simulink model "player_ball_7_8players3_2_withoutlidar"  (R2021b)
settings: Solver=VariableStepAuto  StartTime=0.0  StopTime=300  RelTol=1e-3
model workspace (MAT data in the model file):
  trailfuzzy = 'trailfuzzy.fis'
values from neighbouring files (symbols this model uses):
  initBallPos = fieldCenter    [robotSoccerParams.m]
  robotDetectorMaxHits = 5    [robotSoccerParams.m]
  sampleTime = 0.05    [robotSoccerParams.m]
undefined symbols (not defined in the file or in its folder): DiscIntNeverNeededParam
libraries: mobileRoboticsLib x45, dspindex x15, fuzblock x9
(part 1 of 2)
settings Model: NumberOfSteps=10  Creator=kstkr  LastModifiedBy=kstkr
settings DebuggingCC: AlgebraicLoopMsg=none

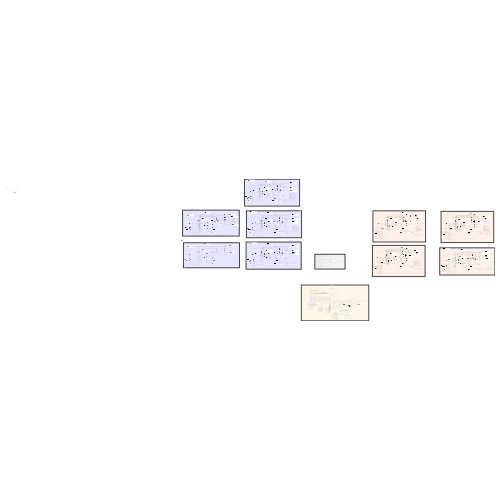
[thumbnail: Simulink's stored preview of the top-level diagram]
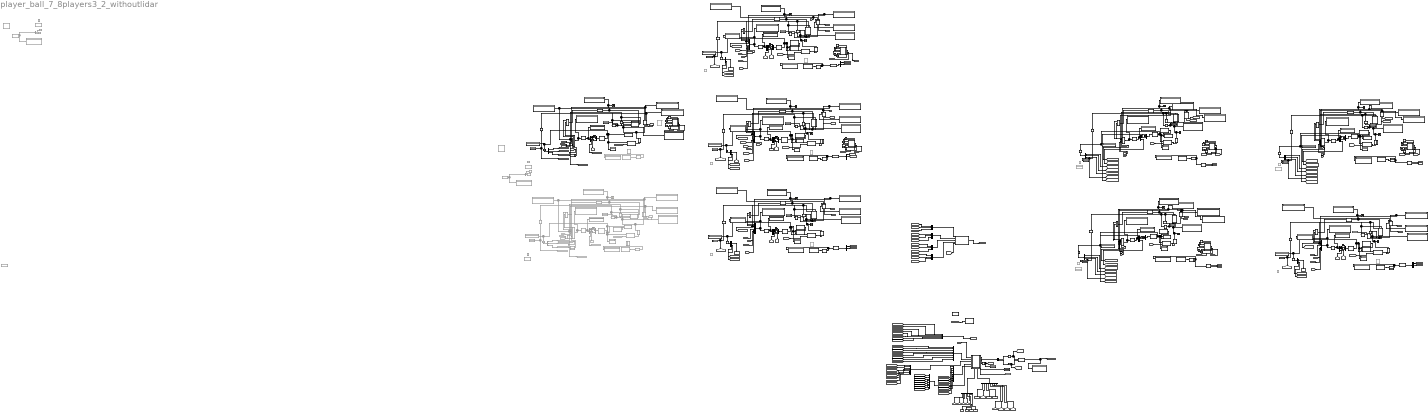
== system player_ball_7_8players3_2_withoutlidar ==
  note: EMOTIONS
  note: Subsystem1
  note: Subsystem1
  note: Ensure the sensor parameters point to the same variables.
  note: Checks team possession and ball held
  note: change mf to sinesoidal
  note: check for postition 80,10
  note: Subsystem1
  note: change mf to sinesoidal
  note: check for postition 80,10
  note: Subsystem1
  note: Ensure the sensor parameters point to the same variables.
  note: Attackert2_1
  note: Ensure the sensor parameters point to the same variables.
  note: Attackert2_2
  note: Ensure the sensor parameters point to the same variables.
  note: defendert2
  note: Ensure the sensor parameters point to the same variables.
  note: Subsystem1
  note: Ensure the sensor parameters point to the same variables.
  note: defentert2_1
  note: Ensure the sensor parameters point to the same variables.
  Add Constant{,1..3} (4 alike) : Bias  Commented=on  Bias=0.3
  Ball Dynamics : MATLAB Function  Commented=on  TreatAsAtomicUnit=on
  Ball Dynamics1 : MATLAB Function  Commented=on  TreatAsAtomicUnit=on
  Ball Dynamics2 : MATLAB Function  Commented=on  TreatAsAtomicUnit=on
  Ball Dynamics3 : MATLAB Function  Commented=on  TreatAsAtomicUnit=on
  Ball Dynamics4 : MATLAB Function  Commented=on  TreatAsAtomicUnit=on
  Ball Dynamics5 : MATLAB Function  Commented=on  TreatAsAtomicUnit=on
  Ball Dynamics6 : MATLAB Function  Commented=on  TreatAsAtomicUnit=on
  Bus Creator{,1..6} (7 alike) : BusCreator  Inputs=8
  Chart3 : Stateflow chart  TreatAsAtomicUnit=on
      settings: PortSchema="{\"entries\":[{\"content\":{\"sides\":[{\"content\":{\"connectorIds\":[\"In1\",\"In2\",\"In3\",\"In4\",\"In6\"]},\"type\":\"ConnectorPlacement.EquallySpacedRectSide\",\"uuid\":\"100227f9-96df-4219-ace2-0d84d12d506e\"},{\"content\":{\"connectorIds\":[\"Out1\",\"Out2\",\"Out3\",\"Out4\"],\"side\":\"RIGHT\"},\"type\":\"ConnectorPlacement.EquallySpacedRectSide\",\"uuid\":\"5179a9f1-5caf-4bf7-8381-53191773d399\"},{\"content\":{\"connectorIds\":[],\"side\":\"TOP\"},\"type\":\"ConnectorPlacement.EquallySpacedRectSide\",\"uuid\":\"b02881a3-df96-4ac6-93d3-ffe2a0056366\"},{\"content\":{\"connectorIds\":[\"In7\",\"In5\"],\"side\":\"BOTTOM\"},\"type\":\"ConnectorPlacement.EquallySpacedRectSide\",\"uuid\":\"6df5f698-3dd3-4c11-801f-bca33302808b\"}]},\"type\":\"ConnectorPlacement.EquallySpacedConnector\",\"uuid\":\"a5fc3484-c51e-4d4d-931a-fb20b747c02a\"}],\"packageUris\":[\"http://schema.mathworks.com/mf0/Connector/R2020b\"],\"version\":\"1.0\"}"
  Constant{,1..9} (10 alike) : Constant  Commented=on  Value=0.5
  Demux{,2,6..10,12..24,26..33} (28 alike) : Demux  Outputs=3
  Demux1 : Demux  Commented=on  Outputs=3
  Demux11 : Demux  Outputs=2
  Demux25 : Demux  Commented=on  Outputs=2
  Demux3 : Demux  Commented=on  Outputs=3
  Demux4 : Demux  Commented=on  Outputs=2
  Demux5 : Demux  Commented=on  Outputs=3
  Display{,1,3,6..9,11,13..24,31..41,43..96} (85 alike) : Display
  Display{2,4..5,10,12,25..30,42} (12 alike) : Display  Commented=on
  From29 : From  Commented=on  GotoTag=objPoses
  From30 : From  Commented=on  GotoTag=rPose_y3
  From31 : From  Commented=on  GotoTag=rPose_theta3
  From32 : From  Commented=on  GotoTag=rPose_y3
  From33 : From  Commented=on  GotoTag=teamHeld
  From34 : From  Commented=on  GotoTag=rPose_x3
  From35 : From  Commented=on  GotoTag=rPose_x3
  Generic Vehicle Simulation : mobileRoboticsLib/Utilities/Generic Vehicle Simulation  initX=25  initY=28  initAngle=0  Ts=sampleTime
      settings: SourceProductName=Mobile Robotics Simulation Toolbox
  Generic Vehicle Simulation1 : mobileRoboticsLib/Utilities/Generic Vehicle Simulation  Commented=on  initX=30  initY=50  initAngle=0  Ts=sampleTime
      settings: SourceProductName=Mobile Robotics Simulation Toolbox
  Generic Vehicle Simulation2 : mobileRoboticsLib/Utilities/Generic Vehicle Simulation  initX=25  initY=15  initAngle=0  Ts=sampleTime
      settings: SourceProductName=Mobile Robotics Simulation Toolbox
  Generic Vehicle Simulation3 : mobileRoboticsLib/Utilities/Generic Vehicle Simulation  initX=2  initY=30  initAngle=0  Ts=sampleTime
      settings: SourceProductName=Mobile Robotics Simulation Toolbox
  Generic Vehicle Simulation4 : mobileRoboticsLib/Utilities/Generic Vehicle Simulation  initX=60  initY=40  initAngle=pi  Ts=sampleTime
      settings: SourceProductName=Mobile Robotics Simulation Library
  Generic Vehicle Simulation5 : mobileRoboticsLib/Utilities/Generic Vehicle Simulation  initX=60  initY=20  initAngle=pi  Ts=sampleTime
      settings: SourceProductName=Mobile Robotics Simulation Library
  Generic Vehicle Simulation6 : mobileRoboticsLib/Utilities/Generic Vehicle Simulation  initX=75  initY=30  initAngle=pi  Ts=sampleTime
      settings: SourceProductName=Mobile Robotics Simulation Library
  Generic Vehicle Simulation7 : mobileRoboticsLib/Utilities/Generic Vehicle Simulation  initX=88  initY=30  initAngle=pi  Ts=sampleTime
      settings: SourceProductName=Mobile Robotics Simulation Toolbox
  Generic Vehicle Simulation8 : mobileRoboticsLib/Utilities/Generic Vehicle Simulation  initX=15  initY=45  initAngle=0  Ts=sampleTime
      settings: SourceProductName=Mobile Robotics Simulation Toolbox
  Goal Range{,1,3..5} (5 alike) : Display
  Goal Range2 : Display  Commented=on
  GoalLeftAngle{,1,3..5} (5 alike) : Display
  GoalLeftAngle2 : Display  Commented=on
  Goto19 : Goto  Commented=on  GotoTag=ballHeld3
  Goto20 : Goto  Commented=on  GotoTag=KickPower3
  Goto21 : Goto  Commented=on  GotoTag=rPose_x3
  Goto22 : Goto  Commented=on  GotoTag=rPose_y3
  Goto23 : Goto  Commented=on  GotoTag=rPose_theta3
  Goto24 : Goto  Commented=on  GotoTag=robotIdx3
  Goto25 : Goto  Commented=on  GotoTag=ballVel3
  Ground{,2..8} (8 alike) : Ground
  Ground1 : Ground  Commented=on
  IC{1,4,10,13,16,19,22,25} (8 alike) : InitialCondition
  IC{2..3,5..6,11..12,14..15,17..18,20..21,23..24,26..27} (16 alike) : InitialCondition  Value=0
  IC7 : InitialCondition  Commented=on
  IC8 : InitialCondition  Commented=on  Value=0
  IC9 : InitialCondition  Commented=on  Value=0
  MATLAB Function : MATLAB Function  TreatAsAtomicUnit=on
  MATLAB Function1 : MATLAB Function  Commented=on  TreatAsAtomicUnit=on
  MATLAB Function10 : MATLAB Function  TreatAsAtomicUnit=on
  MATLAB Function11 : MATLAB Function  TreatAsAtomicUnit=on
  MATLAB Function12 : MATLAB Function  TreatAsAtomicUnit=on
  MATLAB Function2 : MATLAB Function  TreatAsAtomicUnit=on
  MATLAB Function3 : MATLAB Function  Commented=on  TreatAsAtomicUnit=on
  MATLAB Function4 : MATLAB Function  TreatAsAtomicUnit=on
  MATLAB Function5 : MATLAB Function  TreatAsAtomicUnit=on
  MATLAB Function6 : MATLAB Function  TreatAsAtomicUnit=on
  MATLAB Function7 : MATLAB Function  TreatAsAtomicUnit=on
  MATLAB Function8 : MATLAB Function  TreatAsAtomicUnit=on
  MATLAB Function9 : MATLAB Function  TreatAsAtomicUnit=on
  Memory{,3..4,7..11} (8 alike) : Memory  InitialCondition=[15 2 0]  InheritSampleTime=on
  Memory1 : Memory  InheritSampleTime=on
  Memory{12,16,20,24,28,32} (6 alike) : Memory  InitialCondition=5  InheritSampleTime=on
  Memory{13,15,17,19,21,23,25,27,29,31,33,35} (12 alike) : Memory  InitialCondition=2  InheritSampleTime=on
  Memory{14,18,22,26,30,34} (6 alike) : Memory  InitialCondition=8  InheritSampleTime=on
  Memory2 : Memory  Commented=on  InitialCondition=[15 2 0]  InheritSampleTime=on
  Memory5 : Memory  InheritSampleTime=on  LinearizeAsDelay=on
  Memory6 : Memory  InheritSampleTime=on  LinearizeAsDelay=on
  Multi-Robot Environment : mobileRoboticsLib/Environments/Multi-Robot Environment  numRobots=8  mapName=map  showWaypoints=off  showObjects=on  objectColors=objColors  objectMarkers=objMarkers  showRobotIds=on  plotSensorLines=on
      settings: SourceProductName=Mobile Robotics Simulation Toolbox
  Multi-Robot Lidar Sensor2 : mobileRoboticsLib/Environments/Multi-Robot Lidar Sensor  robotIdx=2  mapName=map  sensorOffset=[0,0]  scanAngles=[-pi/4 0 pi/4]  maxRange=5
      settings: SourceProductName=Mobile Robotics Simulation Toolbox
  Multi-Robot Lidar Sensor3 : mobileRoboticsLib/Environments/Multi-Robot Lidar Sensor  Commented=on  robotIdx=3  mapName=map  sensorOffset=[0,0]  scanAngles=[-pi/4 0 pi/4]  maxRange=5
      settings: SourceProductName=Mobile Robotics Simulation Toolbox
  Multi-Robot Lidar Sensor4 : mobileRoboticsLib/Environments/Multi-Robot Lidar Sensor  robotIdx=4  mapName=map  sensorOffset=[0,0]  scanAngles=[-pi/4 0 pi/4]  maxRange=5
      settings: SourceProductName=Mobile Robotics Simulation Toolbox
  Multi-Robot Lidar Sensor5 : mobileRoboticsLib/Environments/Multi-Robot Lidar Sensor  robotIdx=5  mapName=map  sensorOffset=[0,0]  scanAngles=[-pi/4 0 pi/4]  maxRange=5
      settings: SourceProductName=Mobile Robotics Simulation Toolbox
  Multi-Robot Lidar Sensor6 : mobileRoboticsLib/Environments/Multi-Robot Lidar Sensor  robotIdx=6  mapName=map  sensorOffset=[0,0]  scanAngles=[-pi/4 0 pi/4]  maxRange=5
      settings: SourceProductName=Mobile Robotics Simulation Toolbox
  Multi-Robot Lidar Sensor7 : mobileRoboticsLib/Environments/Multi-Robot Lidar Sensor  robotIdx=7  mapName=map  sensorOffset=[0,0]  scanAngles=[-pi/4 0 pi/4]  maxRange=5
      settings: SourceProductName=Mobile Robotics Simulation Toolbox
  Multi-Robot Lidar Sensor8 : mobileRoboticsLib/Environments/Multi-Robot Lidar Sensor  robotIdx=8  mapName=map  sensorOffset=[0,0]  scanAngles=[-pi/4 0 pi/4]  maxRange=5
      settings: SourceProductName=Mobile Robotics Simulation Toolbox
  Multi-Robot Lidar Sensor9 : mobileRoboticsLib/Environments/Multi-Robot Lidar Sensor  robotIdx=3  mapName=map  sensorOffset=[0,0]  scanAngles=[-pi/4 0 pi/4]  maxRange=5
      settings: SourceProductName=Mobile Robotics Simulation Toolbox
  Multi-Robot Visualizer : mobileRoboticsLib/Environments/Multi-Robot Visualizer  idx=1  radius=1  robotColor=[0 0 1]  showTraj=on  hasLidar=off  sensorOffset=[0,0]  scanAngles=[-pi/4 0 pi/4]  maxNumScans=0  hasObjDetector=off  objDetectorOffset=[0,0]  objDetectorAngle=0  objDetectorFOV=pi/3  objDetectorMaxRange=5  hasRobotDetector=off  robotDetectorOffset=[0,0]  robotDetectorAngle=0  robotDetectorFOV=pi/3  robotDetectorMaxRange=5  robotDetectorNumDetections=0
      settings: SourceProductName=Mobile Robotics Simulation Toolbox
  Multi-Robot Visualizer1 : mobileRoboticsLib/Environments/Multi-Robot Visualizer  Commented=on  idx=3  radius=1  robotColor=[0 0 1]  showTraj=on  hasLidar=on  sensorOffset=[0,0]  scanAngles=[-pi/4 0 pi/4]  maxNumScans=0  hasObjDetector=off  objDetectorOffset=[0,0]  objDetectorAngle=0  objDetectorFOV=pi/3  objDetectorMaxRange=5  hasRobotDetector=off  robotDetectorOffset=[0,0]  robotDetectorAngle=0  robotDetectorFOV=pi/3  robotDetectorMaxRange=5  robotDetectorNumDetections=0
      settings: SourceProductName=Mobile Robotics Simulation Toolbox
  Multi-Robot Visualizer2 : mobileRoboticsLib/Environments/Multi-Robot Visualizer  idx=2  radius=1  robotColor=[0 0 1]  showTraj=on  hasLidar=on  sensorOffset=[0,0]  scanAngles=[-pi/4 0 pi/4]  maxNumScans=0  hasObjDetector=off  objDetectorOffset=[0,0]  objDetectorAngle=0  objDetectorFOV=pi/3  objDetectorMaxRange=5  hasRobotDetector=off  robotDetectorOffset=[0,0]  robotDetectorAngle=0  robotDetectorFOV=pi/3  robotDetectorMaxRange=5  robotDetectorNumDetections=0
      settings: SourceProductName=Mobile Robotics Simulation Toolbox
  Multi-Robot Visualizer3 : mobileRoboticsLib/Environments/Multi-Robot Visualizer  idx=4  radius=1  robotColor=[0 0 1]  showTraj=on  hasLidar=on  sensorOffset=[0,0]  scanAngles=[-pi/4 0 pi/4]  maxNumScans=0  hasObjDetector=off  objDetectorOffset=[0,0]  objDetectorAngle=0  objDetectorFOV=pi/3  objDetectorMaxRange=5  hasRobotDetector=off  robotDetectorOffset=[0,0]  robotDetectorAngle=0  robotDetectorFOV=pi/3  robotDetectorMaxRange=5  robotDetectorNumDetections=0
      settings: SourceProductName=Mobile Robotics Simulation Toolbox
  Multi-Robot Visualizer4 : mobileRoboticsLib/Environments/Multi-Robot Visualizer  idx=5  radius=1  robotColor=[1 0 0]  showTraj=on  hasLidar=on  sensorOffset=[0,0]  scanAngles=[-pi/4 0 pi/4]  maxNumScans=0  hasObjDetector=off  objDetectorOffset=[0,0]  objDetectorAngle=0  objDetectorFOV=pi/3  objDetectorMaxRange=5  hasRobotDetector=off  robotDetectorOffset=[0,0]  robotDetectorAngle=0  robotDetectorFOV=pi/3  robotDetectorMaxRange=5  robotDetectorNumDetections=0
      settings: SourceProductName=Mobile Robotics Simulation Toolbox
  Multi-Robot Visualizer5 : mobileRoboticsLib/Environments/Multi-Robot Visualizer  idx=6  radius=1  robotColor=[1 0 0]  showTraj=on  hasLidar=on  sensorOffset=[0,0]  scanAngles=[-pi/4 0 pi/4]  maxNumScans=0  hasObjDetector=off  objDetectorOffset=[0,0]  objDetectorAngle=0  objDetectorFOV=pi/3  objDetectorMaxRange=5  hasRobotDetector=off  robotDetectorOffset=[0,0]  robotDetectorAngle=0  robotDetectorFOV=pi/3  robotDetectorMaxRange=5  robotDetectorNumDetections=0
      settings: SourceProductName=Mobile Robotics Simulation Toolbox
  Multi-Robot Visualizer6 : mobileRoboticsLib/Environments/Multi-Robot Visualizer  idx=7  radius=1  robotColor=[1 0 0]  showTraj=on  hasLidar=on  sensorOffset=[0,0]  scanAngles=[-pi/4 0 pi/4]  maxNumScans=0  hasObjDetector=off  objDetectorOffset=[0,0]  objDetectorAngle=0  objDetectorFOV=pi/3  objDetectorMaxRange=5  hasRobotDetector=off  robotDetectorOffset=[0,0]  robotDetectorAngle=0  robotDetectorFOV=pi/3  robotDetectorMaxRange=5  robotDetectorNumDetections=0
      settings: SourceProductName=Mobile Robotics Simulation Toolbox
  Multi-Robot Visualizer7 : mobileRoboticsLib/Environments/Multi-Robot Visualizer  idx=8  radius=1  robotColor=[1 0 0]  showTraj=on  hasLidar=on  sensorOffset=[0,0]  scanAngles=[-pi/4 0 pi/4]  maxNumScans=0  hasObjDetector=off  objDetectorOffset=[0,0]  objDetectorAngle=0  objDetectorFOV=pi/3  objDetectorMaxRange=5  hasRobotDetector=off  robotDetectorOffset=[0,0]  robotDetectorAngle=0  robotDetectorFOV=pi/3  robotDetectorMaxRange=5  robotDetectorNumDetections=0
      settings: SourceProductName=Mobile Robotics Simulation Toolbox
  Multi-Robot Visualizer8 : mobileRoboticsLib/Environments/Multi-Robot Visualizer  idx=3  radius=1  robotColor=[0 0 1]  showTraj=on  hasLidar=on  sensorOffset=[0,0]  scanAngles=[-pi/4 0 pi/4]  maxNumScans=0  hasObjDetector=off  objDetectorOffset=[0,0]  objDetectorAngle=0  objDetectorFOV=pi/3  objDetectorMaxRange=5  hasRobotDetector=off  robotDetectorOffset=[0,0]  robotDetectorAngle=0  robotDetectorFOV=pi/3  robotDetectorMaxRange=5  robotDetectorNumDetections=0
      settings: SourceProductName=Mobile Robotics Simulation Toolbox
  Mux{,4,6,8,10,12,14,16,18..21} (12 alike) : Mux  Inputs=3
  Mux1 : Mux  Commented=on  Inputs=3
  Mux11 : Mux  Inputs=9
  Mux13 : Mux  Inputs=9
  Mux15 : Mux  Inputs=8
  Mux17 : Mux  Inputs=10
  Mux2 : Mux  Inputs=10
  Mux3 : Mux  Commented=on  Inputs=10
  Mux5 : Mux  Inputs=10
  Mux7 : Mux  Inputs=8
  Mux9 : Mux  Inputs=9
  Object Detections [range, angle, label]{,2..8} (8 alike) : Display
  "Object Detections [range, angle, label]1" : Display  Commented=on
  Object Detector{,2..8} (8 alike) : mobileRoboticsLib/Environments/Object Detector  mapName=map  sensorOffset=objDetectorOffset  sensorAngle=objDetectorAngle  fieldOfView=objDetectorFOV  maxRange=objDetectorRange  maxDetections=objDetectorMaxHits  sampleTime=-1
      Object Detector settings: SourceProductName=Mobile Robotics Simulation Toolbox
      Object Detector2 settings: SourceProductName=Mobile Robotics Simulation Toolbox
      Object Detector3 settings: SourceProductName=Mobile Robotics Simulation Toolbox
      Object Detector4 settings: SourceProductName=Ground Vehicles Library
      Object Detector5 settings: SourceProductName=Ground Vehicles Library
      Object Detector6 settings: SourceProductName=Ground Vehicles Library
      Object Detector7 settings: SourceProductName=Mobile Robotics Simulation Toolbox
      Object Detector8 settings: SourceProductName=Mobile Robotics Simulation Toolbox
  Object Detector1 : mobileRoboticsLib/Environments/Object Detector  Commented=on  mapName=map  sensorOffset=objDetectorOffset  sensorAngle=objDetectorAngle  fieldOfView=objDetectorFOV  maxRange=objDetectorRange  maxDetections=objDetectorMaxHits  sampleTime=-1
      settings: SourceProductName=Mobile Robotics Simulation Toolbox
  "Objects [x, y, label]1" : Constant  Commented=on  Value=[45, 30, 1; 0,15,2; 0, 45, 2; 90, 15, 3; 90, 45, 3]
  "Objects [x, y, label]2" : Constant  Commented=on  Value=[45, 30, 1; 0,15,2; 0, 45, 2; 90, 15, 3; 90, 45, 3]
  Package Objects Array1 : Subsystem
  Plot Soccer Field : MATLAB Function  TreatAsAtomicUnit=on
  Robot Detector1 : mobileRoboticsLib/Environments/Robot Detector  Commented=on  mapName=map  robotIdx=1  sensorOffset=robotDetectorOffset  sensorAngle=robotDetectorAngle  sensorFOV=2*pi  maxRange=100  maxDetections=robotDetectorMaxHits  sampleTime=sampleTime
      link override Robot Detector: mapName=map  maxDetections=5
      settings: SourceProductName=Mobile Robotics Simulation Toolbox
  Robot Detector2 : mobileRoboticsLib/Environments/Robot Detector  mapName=map  robotIdx=2  sensorOffset=robotDetectorOffset  sensorAngle=robotDetectorAngle  sensorFOV=2*pi  maxRange=100  maxDetections=robotDetectorMaxHits  sampleTime=sampleTime
      link override Robot Detector: mapName=map  maxDetections=5
      settings: SourceProductName=Mobile Robotics Simulation Toolbox
  Robot Detector3 : mobileRoboticsLib/Environments/Robot Detector  Commented=on  mapName=map  robotIdx=3  sensorOffset=robotDetectorOffset  sensorAngle=robotDetectorAngle  sensorFOV=2*pi  maxRange=100  maxDetections=robotDetectorMaxHits  sampleTime=sampleTime
      link override Robot Detector: mapName=map  maxDetections=5
      settings: SourceProductName=Mobile Robotics Simulation Toolbox
  Robot Detector4 : mobileRoboticsLib/Environments/Robot Detector  mapName=map  robotIdx=4  sensorOffset=robotDetectorOffset  sensorAngle=robotDetectorAngle  sensorFOV=2*pi  maxRange=100  maxDetections=robotDetectorMaxHits  sampleTime=sampleTime
      link override Robot Detector: mapName=map  maxDetections=5
      settings: SourceProductName=Mobile Robotics Simulation Toolbox
  Robot Detector5 : mobileRoboticsLib/Environments/Robot Detector  mapName=map  robotIdx=5  sensorOffset=robotDetectorOffset  sensorAngle=robotDetectorAngle  sensorFOV=pi/3  maxRange=100  maxDetections=robotDetectorMaxHits  sampleTime=sampleTime
      link override Robot Detector: mapName=map  maxDetections=5
      settings: SourceProductName=Mobile Robotics Simulation Toolbox
  Robot Detector6 : mobileRoboticsLib/Environments/Robot Detector  mapName=map  robotIdx=6  sensorOffset=robotDetectorOffset  sensorAngle=robotDetectorAngle  sensorFOV=pi/3  maxRange=100  maxDetections=robotDetectorMaxHits  sampleTime=sampleTime
      link override Robot Detector: mapName=map  maxDetections=5
      settings: SourceProductName=Mobile Robotics Simulation Toolbox
  Robot Detector7 : mobileRoboticsLib/Environments/Robot Detector  mapName=map  robotIdx=7  sensorOffset=robotDetectorOffset  sensorAngle=robotDetectorAngle  sensorFOV=pi/3  maxRange=100  maxDetections=robotDetectorMaxHits  sampleTime=sampleTime
      link override Robot Detector: mapName=map  maxDetections=5
      settings: SourceProductName=Mobile Robotics Simulation Toolbox
  Robot Detector8 : mobileRoboticsLib/Environments/Robot Detector  mapName=map  robotIdx=8  sensorOffset=robotDetectorOffset  sensorAngle=robotDetectorAngle  sensorFOV=2*pi  maxRange=100  maxDetections=robotDetectorMaxHits  sampleTime=sampleTime
      link override Robot Detector: mapName=map  maxDetections=5
      settings: SourceProductName=Mobile Robotics Simulation Toolbox
  Robot Detector9 : mobileRoboticsLib/Environments/Robot Detector  mapName=map  robotIdx=3  sensorOffset=robotDetectorOffset  sensorAngle=robotDetectorAngle  sensorFOV=2*pi  maxRange=100  maxDetections=robotDetectorMaxHits  sampleTime=sampleTime
      link override Robot Detector: mapName=map  maxDetections=5
      settings: SourceProductName=Mobile Robotics Simulation Toolbox
  Scope{,1,4,6,8,10,12,14} (8 alike) : Scope
  Scope{3,5,7,9,11,13,15} (7 alike) : Scope  NumInputPorts=2
  Scope2 : Scope  Commented=on
  Variable Selector{,3..8,10..14} (12 alike) : dspindex/Variable Selector  NumInputs=1  rowsOrCols=Rows  IdxMode=Fixed  Elements="[1  ]"  ZerOneIdxMode=One-based  errmode=Clip Index  FillMode=off  FillValues=0
  Variable Selector1 : dspindex/Variable Selector  Commented=on  NumInputs=1  rowsOrCols=Rows  IdxMode=Fixed  Elements="[1  ]"  ZerOneIdxMode=One-based  errmode=Clip Index  FillMode=off  FillValues=0
  Variable Selector2 : dspindex/Variable Selector  Commented=on  NumInputs=1  rowsOrCols=Columns  IdxMode=Fixed  Elements=[1 2]  ZerOneIdxMode=One-based  errmode=Clip Index  FillMode=on  FillValues=0
  Variable Selector9 : dspindex/Variable Selector  Commented=on  NumInputs=1  rowsOrCols=Columns  IdxMode=Fixed  Elements=[1 2]  ZerOneIdxMode=One-based  errmode=Clip Index  FillMode=on  FillValues=0
  Zero Pad Detections1 : MATLAB Function  Commented=on  TreatAsAtomicUnit=on  mask(Zero Pad Detections){maxHits=robotDetectorMaxHits}
      mask prompts: maxHits "Maximum Sensor Hits"
      mask help: Zero pads detections matrix so it is fixed-size and works with arrays of buses.
  Zero Pad Detections10 : MATLAB Function  TreatAsAtomicUnit=on  mask(Zero Pad Detections){maxHits=robotDetectorMaxHits}
      mask prompts: maxHits "Maximum Sensor Hits"
      mask help: Zero pads detections matrix so it is fixed-size and works with arrays of buses.
  Zero Pad Detections11 : MATLAB Function  Commented=on  TreatAsAtomicUnit=on  mask(Zero Pad Detections){maxHits=robotDetectorMaxHits}
      mask prompts: maxHits "Maximum Sensor Hits"
      mask help: Zero pads detections matrix so it is fixed-size and works with arrays of buses.
  Zero Pad Detections12 : MATLAB Function  TreatAsAtomicUnit=on  mask(Zero Pad Detections){maxHits=robotDetectorMaxHits}
      mask prompts: maxHits "Maximum Sensor Hits"
      mask help: Zero pads detections matrix so it is fixed-size and works with arrays of buses.
  Zero Pad Detections13 : MATLAB Function  TreatAsAtomicUnit=on  mask(Zero Pad Detections){maxHits=robotDetectorMaxHits}
      mask prompts: maxHits "Maximum Sensor Hits"
      mask help: Zero pads detections matrix so it is fixed-size and works with arrays of buses.
  Zero Pad Detections14 : MATLAB Function  TreatAsAtomicUnit=on  mask(Zero Pad Detections){maxHits=robotDetectorMaxHits}
      mask prompts: maxHits "Maximum Sensor Hits"
      mask help: Zero pads detections matrix so it is fixed-size and works with arrays of buses.
  Zero Pad Detections15 : MATLAB Function  TreatAsAtomicUnit=on  mask(Zero Pad Detections){maxHits=robotDetectorMaxHits}
      mask prompts: maxHits "Maximum Sensor Hits"
      mask help: Zero pads detections matrix so it is fixed-size and works with arrays of buses.
  Zero Pad Detections16 : MATLAB Function  TreatAsAtomicUnit=on  mask(Zero Pad Detections){maxHits=robotDetectorMaxHits}
      mask prompts: maxHits "Maximum Sensor Hits"
      mask help: Zero pads detections matrix so it is fixed-size and works with arrays of buses.
  Zero Pad Detections17 : MATLAB Function  TreatAsAtomicUnit=on  mask(Zero Pad Detections){maxHits=robotDetectorMaxHits}
      mask prompts: maxHits "Maximum Sensor Hits"
      mask help: Zero pads detections matrix so it is fixed-size and works with arrays of buses.
  Zero Pad Detections18 : MATLAB Function  TreatAsAtomicUnit=on  mask(Zero Pad Detections){maxHits=robotDetectorMaxHits}
      mask prompts: maxHits "Maximum Sensor Hits"
      mask help: Zero pads detections matrix so it is fixed-size and works with arrays of buses.
  Zero Pad Detections19 : MATLAB Function  TreatAsAtomicUnit=on  mask(Zero Pad Detections){maxHits=robotDetectorMaxHits}
      mask prompts: maxHits "Maximum Sensor Hits"
      mask help: Zero pads detections matrix so it is fixed-size and works with arrays of buses.
  Zero Pad Detections2 : MATLAB Function  Commented=on  TreatAsAtomicUnit=on  mask(Zero Pad Detections){maxHits=robotDetectorMaxHits}
      mask prompts: maxHits "Maximum Sensor Hits"
      mask help: Zero pads detections matrix so it is fixed-size and works with arrays of buses.
  Zero Pad Detections20 : MATLAB Function  Commented=on  TreatAsAtomicUnit=on  mask(Zero Pad Detections){maxHits=robotDetectorMaxHits}
      mask prompts: maxHits "Maximum Sensor Hits"
      mask help: Zero pads detections matrix so it is fixed-size and works with arrays of buses.
  Zero Pad Detections21 : MATLAB Function  TreatAsAtomicUnit=on  mask(Zero Pad Detections){maxHits=robotDetectorMaxHits}
      mask prompts: maxHits "Maximum Sensor Hits"
      mask help: Zero pads detections matrix so it is fixed-size and works with arrays of buses.
  Zero Pad Detections22 : MATLAB Function  TreatAsAtomicUnit=on  mask(Zero Pad Detections){maxHits=robotDetectorMaxHits}
      mask prompts: maxHits "Maximum Sensor Hits"
      mask help: Zero pads detections matrix so it is fixed-size and works with arrays of buses.
  Zero Pad Detections23 : MATLAB Function  Commented=on  TreatAsAtomicUnit=on  mask(Zero Pad Detections){maxHits=robotDetectorMaxHits}
      mask prompts: maxHits "Maximum Sensor Hits"
      mask help: Zero pads detections matrix so it is fixed-size and works with arrays of buses.
  Zero Pad Detections24 : MATLAB Function  TreatAsAtomicUnit=on  mask(Zero Pad Detections){maxHits=robotDetectorMaxHits}
      mask prompts: maxHits "Maximum Sensor Hits"
      mask help: Zero pads detections matrix so it is fixed-size and works with arrays of buses.
  Zero Pad Detections3 : MATLAB Function  Commented=on  TreatAsAtomicUnit=on  mask(Zero Pad Detections){maxHits=robotDetectorMaxHits}
      mask prompts: maxHits "Maximum Sensor Hits"
      mask help: Zero pads detections matrix so it is fixed-size and works with arrays of buses.
  Zero Pad Detections4 : MATLAB Function  TreatAsAtomicUnit=on  mask(Zero Pad Detections){maxHits=robotDetectorMaxHits}
      mask prompts: maxHits "Maximum Sensor Hits"
      mask help: Zero pads detections matrix so it is fixed-size and works with arrays of buses.
  Zero Pad Detections5 : MATLAB Function  TreatAsAtomicUnit=on  mask(Zero Pad Detections){maxHits=robotDetectorMaxHits}
      mask prompts: maxHits "Maximum Sensor Hits"
      mask help: Zero pads detections matrix so it is fixed-size and works with arrays of buses.
  Zero Pad Detections6 : MATLAB Function  Commented=on  TreatAsAtomicUnit=on  mask(Zero Pad Detections){maxHits=robotDetectorMaxHits}
      mask prompts: maxHits "Maximum Sensor Hits"
      mask help: Zero pads detections matrix so it is fixed-size and works with arrays of buses.
  Zero Pad Detections7 : MATLAB Function  TreatAsAtomicUnit=on  mask(Zero Pad Detections){maxHits=robotDetectorMaxHits}
      mask prompts: maxHits "Maximum Sensor Hits"
      mask help: Zero pads detections matrix so it is fixed-size and works with arrays of buses.
  Zero Pad Detections8 : MATLAB Function  Commented=on  TreatAsAtomicUnit=on  mask(Zero Pad Detections){maxHits=robotDetectorMaxHits}
      mask prompts: maxHits "Maximum Sensor Hits"
      mask help: Zero pads detections matrix so it is fixed-size and works with arrays of buses.
  Zero Pad Detections9 : MATLAB Function  Commented=on  TreatAsAtomicUnit=on  mask(Zero Pad Detections){maxHits=robotDetectorMaxHits}
      mask prompts: maxHits "Maximum Sensor Hits"
      mask help: Zero pads detections matrix so it is fixed-size and works with arrays of buses.
  ball : MATLAB Function  TreatAsAtomicUnit=on
  ball1 : MATLAB Function  TreatAsAtomicUnit=on
  ball2 : MATLAB Function  TreatAsAtomicUnit=on
  ball3 : MATLAB Function  Commented=on  TreatAsAtomicUnit=on
  ball4 : MATLAB Function  TreatAsAtomicUnit=on
  ball5 : MATLAB Function  TreatAsAtomicUnit=on
  ball6 : MATLAB Function  TreatAsAtomicUnit=on
  ball7 : MATLAB Function  TreatAsAtomicUnit=on
  ball8 : MATLAB Function  TreatAsAtomicUnit=on
  idx3 goal_range_angles : MATLAB Function  TreatAsAtomicUnit=on
  idx3 goal_range_angles1 : MATLAB Function  TreatAsAtomicUnit=on
  idx3 goal_range_angles2 : MATLAB Function  TreatAsAtomicUnit=on
  idx3 goal_range_angles3 : MATLAB Function  Commented=on  TreatAsAtomicUnit=on
  idx3 goal_range_angles4 : MATLAB Function  TreatAsAtomicUnit=on
  idx3 goal_range_angles5 : MATLAB Function  TreatAsAtomicUnit=on
  idx3 goal_range_angles6 : MATLAB Function  TreatAsAtomicUnit=on
  idx3 goal_range_angles7 : MATLAB Function  TreatAsAtomicUnit=on
  idx3 goal_range_angles8 : MATLAB Function  TreatAsAtomicUnit=on
  robot_actions1 : fuzblock/Fuzzy Logic  Controller  FIS='A1trialfuzzyball6_2.fis'  OutputSampleNumber=101  DataType=double  FuzzifiedInputs=off  RuleFiringStrengths=off  RuleOutputs=off  AggregatedOutputs=off  SimulateUsing=Interpreted execution  OutOfRangeInputValueMessage=warning  NoRuleFiredMessage=warning  EmptyOutputFuzzySetMessage=warning
  robot_actions2 : fuzblock/Fuzzy Logic  Controller  Commented=on  FIS='A1trialfuzzyball6_2.fis'  OutputSampleNumber=101  DataType=double  FuzzifiedInputs=off  RuleFiringStrengths=off  RuleOutputs=off  AggregatedOutputs=off  SimulateUsing=Interpreted execution  OutOfRangeInputValueMessage=warning  NoRuleFiredMessage=warning  EmptyOutputFuzzySetMessage=warning
  robot_actions3 : fuzblock/Fuzzy Logic  Controller  FIS='D1trialfuzzyball6_1_1.fis'  OutputSampleNumber=101  DataType=double  FuzzifiedInputs=off  RuleFiringStrengths=off  RuleOutputs=off  AggregatedOutputs=off  SimulateUsing=Interpreted execution  OutOfRangeInputValueMessage=warning  NoRuleFiredMessage=warning  EmptyOutputFuzzySetMessage=warning
  robot_actions4 : fuzblock/Fuzzy Logic  Controller  FIS='G1trialfuzzyball4.fis'  OutputSampleNumber=101  DataType=double  FuzzifiedInputs=off  RuleFiringStrengths=off  RuleOutputs=off  AggregatedOutputs=off  SimulateUsing=Interpreted execution  OutOfRangeInputValueMessage=warning  NoRuleFiredMessage=warning  EmptyOutputFuzzySetMessage=warning
  robot_actions5 : fuzblock/Fuzzy Logic  Controller  FIS='A1trialfuzzyball3_1.fis'  OutputSampleNumber=101  DataType=double  FuzzifiedInputs=off  RuleFiringStrengths=off  RuleOutputs=off  AggregatedOutputs=off  SimulateUsing=Interpreted execution  OutOfRangeInputValueMessage=warning  NoRuleFiredMessage=warning  EmptyOutputFuzzySetMessage=warning
  robot_actions6 : fuzblock/Fuzzy Logic  Controller  FIS='A1trialfuzzyball3_1.fis'  OutputSampleNumber=101  DataType=double  FuzzifiedInputs=off  RuleFiringStrengths=off  RuleOutputs=off  AggregatedOutputs=off  SimulateUsing=Interpreted execution  OutOfRangeInputValueMessage=warning  NoRuleFiredMessage=warning  EmptyOutputFuzzySetMessage=warning
  robot_actions7 : fuzblock/Fuzzy Logic  Controller  FIS='A1trialfuzzyball3_1.fis'  OutputSampleNumber=101  DataType=double  FuzzifiedInputs=off  RuleFiringStrengths=off  RuleOutputs=off  AggregatedOutputs=off  SimulateUsing=Interpreted execution  OutOfRangeInputValueMessage=warning  NoRuleFiredMessage=warning  EmptyOutputFuzzySetMessage=warning
  robot_actions8 : fuzblock/Fuzzy Logic  Controller  FIS='G2trialfuzzyball4.fis'  OutputSampleNumber=101  DataType=double  FuzzifiedInputs=off  RuleFiringStrengths=off  RuleOutputs=off  AggregatedOutputs=off  SimulateUsing=Interpreted execution  OutOfRangeInputValueMessage=warning  NoRuleFiredMessage=warning  EmptyOutputFuzzySetMessage=warning
  robot_actions9 : fuzblock/Fuzzy Logic  Controller  FIS='D1trialfuzzyball6_2_1.fis'  OutputSampleNumber=101  DataType=double  FuzzifiedInputs=off  RuleFiringStrengths=off  RuleOutputs=off  AggregatedOutputs=off  SimulateUsing=Interpreted execution  OutOfRangeInputValueMessage=warning  NoRuleFiredMessage=warning  EmptyOutputFuzzySetMessage=warning
  wires:
  Robot Detector1/1 -> Zero Pad Detections2/1(u)
  Zero Pad Detections2/1(y) -> Display5/1  "robotDetections"
  Mux/1 -> Generic Vehicle Simulation/1
  Ground/1 -> Mux/2
  robot_actions1/1 -> Display13/1, Demux/1  "v"
  Demux/1 -> [ballVel1], Mux/1
  Demux/2 -> Mux/3
  Generic Vehicle Simulation/1 -> Display11/1, Memory/1, Display/1, Object Detector/1, Multi-Robot Visualizer/1  "pose"
  Mux2/1 -> Display3/1, robot_actions1/1
  Object Detector/1 -> Zero Pad Detections4/1(u)  "detections"
  Variable Selector/1 -> Demux2/1
  Demux2/1 -> Mux2/2
  [objPoses] -> Multi-Robot Environment/1
  Demux2/2 -> Mux2/1
  Zero Pad Detections4/1(y) -> ball/1(u), "Object Detections [range, angle, label]"/1, idx3 goal_range_angles/1(u)  "robotDetections"
  ball/1(y) -> Scope/1, Display9/1, Variable Selector/1
  idx3 goal_range_angles/1(goalRight_angle) -> Mux2/4, Display6/1
  idx3 goal_range_angles/2(goalRange) -> Goal Range/1, Mux2/5
  idx3 goal_range_angles/3(goalLeft_angle) -> Mux2/6, GoalLeftAngle/1
  Variable Selector2/1 -> Demux4/1, Display10/1
  Demux4/1 -> Add Constant/1
  Demux4/2 -> Add Constant1/1
  Memory/1 -> Demux6/1
  Demux6/1 -> [rPose_x1]
  Demux6/2 -> [rPose_y1]
  Demux6/3 -> [rPose_theta1]
  Demux/3 -> [KickPower1]
  ball/3(robotIdx) -> IC1/1, IC2/1
  IC1/1 -> [robotIdx1], Display15/1
  ball/2(ballHeld) -> [ballHeld1], Mux2/3, IC3/1
  IC2/1 -> Display14/1, ball/3("robotIdx ")
  IC3/1 -> ball/2("ballHeld ")
  IC6/1 -> Display18/1, ball1/2("ballHeld ")
  IC5/1 -> ball1/3("robotIdx ")
  ball1/2(ballHeld) -> IC6/1, [ballHeld2], Mux5/3
  IC4/1 -> Display19/1, [robotIdx2]
  ball1/3(robotIdx) -> IC5/1, IC4/1
  Demux7/3 -> [KickPower2]
  Demux10/3 -> [rPose_theta2]
  Demux10/2 -> [rPose_y2]
  Demux10/1 -> [rPose_x2]
  Memory4/1 -> Demux10/1
  idx3 goal_range_angles1/3(goalLeft_angle) -> GoalLeftAngle1/1
  idx3 goal_range_angles1/2(goalRange) -> Mux5/4, Goal Range1/1
  idx3 goal_range_angles1/1(goalRight_angle) -> [leftpoleangle2], Display22/1
  ball1/1(y) -> Variable Selector3/1, Display23/1, Scope1/1
  Zero Pad Detections7/1(y) -> "Object Detections [range, angle, label]2"/1, ball1/1(u), idx3 goal_range_angles1/1(u), Scope3/1  "robotDetections"
  Demux8/2 -> Mux5/1
  Multi-Robot Lidar Sensor2/1 -> Multi-Robot Visualizer2/2
  Demux8/1 -> Mux5/2
  Variable Selector3/1 -> Demux8/1
  Object Detector2/1 -> Zero Pad Detections7/1(u)  "detections"
  Mux5/1 -> robot_actions3/1, Display16/1, Display20/1
  Generic Vehicle Simulation2/1 -> Multi-Robot Visualizer2/1, Display7/1, Object Detector2/1, Memory4/1, Display8/1  "pose"
  Demux7/2 -> Mux4/3
  Demux7/1 -> [ballVel2], Mux4/1
  robot_actions3/1 -> Demux7/1, Display17/1  "v"
  Ground2/1 -> Mux4/2
  Mux4/1 -> Generic Vehicle Simulation2/1
  Zero Pad Detections5/1(y) -> Variable Selector4/1, Display21/1  "robotDetections"
  Robot Detector2/1 -> Zero Pad Detections5/1(u)
  [objPoses] -> Object Detector/2
  [objPoses] -> Object Detector2/2
  Demux9/2 -> [rdet_angle]
  Demux9/1 -> [rdet_range]
  [rdet_range] -> Mux5/5
  [rdet_angle] -> Mux5/6
  Variable Selector4/1 -> Demux9/1
  Chart3/1(ballPose) -> Demux11/1
  [rPose_theta2] -> Bus Creator6/2
  [rPose_theta1] -> Bus Creator6/1
  [ballVel2] -> Bus Creator5/2
  [ballVel1] -> Bus Creator5/1
  [robotIdx2] -> Bus Creator2/2
  [robotIdx1] -> Bus Creator2/1
  [rPose_y2] -> Bus Creator4/2
  [rPose_y1] -> Bus Creator4/1
  [rPose_x2] -> Bus Creator3/2
  [rPose_x1] -> Bus Creator3/1
  [KickPower2] -> Bus Creator1/2
  [KickPower1] -> Bus Creator1/1
  [ballHeld2] -> Bus Creator/2
  [ballHeld1] -> Bus Creator/1
  Bus Creator6/1 -> Chart3/5(rPose_theta)
  Bus Creator5/1 -> Chart3/7(ballVel)
  Bus Creator4/1 -> Chart3/4(rPose_y)
  Bus Creator3/1 -> Chart3/3(rPose_x)
  Bus Creator2/1 -> Chart3/6(robotIdx)
  Bus Creator1/1 -> Chart3/2(KickPower)
  Bus Creator/1 -> [BALLHELD]
  Package Objects Array1/1(objectsPose) -> Display24/1, [objPoses]
  Memory5/1 -> [ballPose_y], Package Objects Array1/2(In2)
  Memory6/1 -> [ballPose_x], Package Objects Array1/1(Inport)
  Demux11/2 -> Memory5/1
  Demux11/1 -> Memory6/1
  Chart3/2(teamHeld) -> Memory1/1
  [ballPose_x] -> Mux5/7
  [teamHeld] -> Mux5/8
  Memory1/1 -> Display1/1, [teamHeld]
  [teamHeld] -> Mux2/7
  [rPose_x1] -> Mux2/8
  [rPose_x1] -> idx3 goal_range_angles/2(rPose_x)
  [rPose_y1] -> idx3 goal_range_angles/3(rPose_y)
  [rPose_x2] -> idx3 goal_range_angles1/2(rPose_x)
  [rPose_y2] -> idx3 goal_range_angles1/3(rPose_y)
  [rPose_theta1] -> MATLAB Function/1(u)
  [rPose_y1] -> Mux2/10
  MATLAB Function/1(y) -> Mux2/9
  MATLAB Function1/1(y) -> Mux3/9
  From32/1 -> Mux3/10
  From31/1 -> MATLAB Function1/1(u)
  From30/1 -> idx3 goal_range_angles3/3(rPose_y)
  From35/1 -> idx3 goal_range_angles3/2(rPose_x)
  From34/1 -> Mux3/8
  From33/1 -> Mux3/7
  From29/1 -> Object Detector1/2
  IC9/1 -> ball3/2("ballHeld ")
  IC8/1 -> ball3/3("robotIdx "), Display25/1
  ball3/2(ballHeld) -> IC9/1, Mux3/3, Goto19/1
  IC7/1 -> Display26/1, Goto24/1
  ball3/3(robotIdx) -> IC8/1, IC7/1
  Demux1/3 -> Goto20/1
  Demux5/3 -> Goto23/1
  Demux5/2 -> Goto22/1
  Demux5/1 -> Goto21/1
  Memory2/1 -> Demux5/1
  idx3 goal_range_angles3/3(goalLeft_angle) -> GoalLeftAngle2/1, Mux3/6
  idx3 goal_range_angles3/2(goalRange) -> Mux3/5, Goal Range2/1
  idx3 goal_range_angles3/1(goalRight_angle) -> Display29/1, Mux3/4
  ball3/1(y) -> Variable Selector1/1, Display30/1, Scope2/1
  Zero Pad Detections9/1(y) -> idx3 goal_range_angles3/1(u), "Object Detections [range, angle, label]1"/1, ball3/1(u)  "robotDetections"
  Demux3/2 -> Mux3/1
  Multi-Robot Lidar Sensor3/1 -> Multi-Robot Visualizer1/2
  Demux3/1 -> Mux3/2
  Variable Selector1/1 -> Demux3/1
  Object Detector1/1 -> Zero Pad Detections9/1(u)  "detections"
  Mux3/1 -> robot_actions2/1, Display27/1
  Generic Vehicle Simulation1/1 -> Multi-Robot Visualizer1/1, Object Detector1/1, Display2/1, Memory2/1, Display4/1  "pose"
  Demux1/2 -> Mux1/3
  Demux1/1 -> Mux1/1, Goto25/1
  robot_actions2/1 -> Demux1/1, Display12/1  "v"
  Ground1/1 -> Mux1/2
  Mux1/1 -> Generic Vehicle Simulation1/1
  Zero Pad Detections1/1(y) -> Display28/1  "robotDetections"
  Robot Detector3/1 -> Zero Pad Detections1/1(u)
  [rPose_y4] -> idx3 goal_range_angles4/3(rPose_y)
  [rPose_x4] -> idx3 goal_range_angles4/2(rPose_x)
  [teamHeld] -> Mux7/8
  [ballPose_x] -> Mux7/7
  Variable Selector6/1 -> Demux15/1
  [rdet_angle2] -> Mux7/6
  [rdet_range2] -> Mux7/5
  Demux15/1 -> [rdet_range2]
  Demux15/2 -> [rdet_angle2]
  [objPoses] -> Object Detector3/2
  Robot Detector4/1 -> Zero Pad Detections10/1(u)
  Zero Pad Detections10/1(y) -> Display36/1, Variable Selector6/1  "robotDetections"
  Mux6/1 -> Generic Vehicle Simulation3/1
  Ground3/1 -> Mux6/2
  robot_actions4/1 -> Display32/1, Demux13/1  "v"
  Demux13/1 -> Mux6/1, [ballVel4]
  Demux13/2 -> Mux6/3
  Generic Vehicle Simulation3/1 -> Display40/1, Memory3/1, Object Detector3/1, Display39/1, Multi-Robot Visualizer3/1  "pose"
  Mux7/1 -> Display35/1, Display31/1, robot_actions4/1
  Object Detector3/1 -> Zero Pad Detections12/1(u)  "detections"
  Variable Selector5/1 -> Demux14/1
  Demux14/1 -> Mux7/2
  Multi-Robot Lidar Sensor4/1 -> Multi-Robot Visualizer3/2
  Demux14/2 -> Mux7/1
  Zero Pad Detections12/1(y) -> Scope5/1, idx3 goal_range_angles4/1(u), ball4/1(u), "Object Detections [range, angle, label]3"/1  "robotDetections"
  ball4/1(y) -> Scope4/1, Display38/1, Variable Selector5/1
  idx3 goal_range_angles4/1(goalRight_angle) -> Display37/1
  idx3 goal_range_angles4/2(goalRange) -> Goal Range3/1, Mux7/4
  idx3 goal_range_angles4/3(goalLeft_angle) -> GoalLeftAngle3/1
  Memory3/1 -> Demux12/1
  Demux12/1 -> [rPose_x4]
  Demux12/2 -> [rPose_y4]
  Demux12/3 -> [rPose_theta4]
  Demux13/3 -> [KickPower4]
  ball4/3(robotIdx) -> IC10/1, IC11/1
  IC10/1 -> [robotIdx4], Display34/1
  ball4/2(ballHeld) -> Mux7/3, [ballHeld4], IC12/1
  IC11/1 -> ball4/3("robotIdx ")
  IC12/1 -> ball4/2("ballHeld "), Display33/1
  [ballHeld3] -> Bus Creator/3
  [ballHeld4] -> Bus Creator/4
  [KickPower3] -> Bus Creator1/3
  [KickPower4] -> Bus Creator1/4
  [rPose_x3] -> Bus Creator3/3
  [rPose_x4] -> Bus Creator3/4
  [rPose_y3] -> Bus Creator4/3
  [rPose_y4] -> Bus Creator4/4
  [robotIdx3] -> Bus Creator2/3
  [robotIdx4] -> Bus Creator2/4
  [ballVel3] -> Bus Creator5/3
  [ballVel4] -> Bus Creator5/4
  [rPose_theta3] -> Bus Creator6/3
  [rPose_theta4] -> Bus Creator6/4
  Demux25/2 -> Add Constant3/1
  Demux25/1 -> Add Constant2/1
  Variable Selector9/1 -> Display42/1, Demux25/1
  [ballHeld5] -> Bus Creator/5
  [ballHeld6] -> Bus Creator/6
  [ballHeld7] -> Bus Creator/7
  [ballHeld8] -> Bus Creator/8
  [KickPower8] -> Bus Creator1/8
  [KickPower7] -> Bus Creator1/7
  [KickPower5] -> Bus Creator1/5
  [KickPower6] -> Bus Creator1/6
  [rPose_x8] -> Bus Creator3/8
  [rPose_x7] -> Bus Creator3/7
  [rPose_x5] -> Bus Creator3/5
  [rPose_x6] -> Bus Creator3/6
  [rPose_y5] -> Bus Creator4/5
  [rPose_y6] -> Bus Creator4/6
  [rPose_y7] -> Bus Creator4/7
  [rPose_y8] -> Bus Creator4/8
  [robotIdx5] -> Bus Creator2/5
  [robotIdx6] -> Bus Creator2/6
  [robotIdx7] -> Bus Creator2/7
  [robotIdx8] -> Bus Creator2/8
  [ballVel8] -> Bus Creator5/8
  [ballVel7] -> Bus Creator5/7
  [ballVel5] -> Bus Creator5/5
  [ballVel6] -> Bus Creator5/6
  [rPose_theta8] -> Bus Creator6/8
  [rPose_theta7] -> Bus Creator6/7
  [rPose_theta5] -> Bus Creator6/5
  [rPose_theta6] -> Bus Creator6/6
  IC15/1 -> ball2/2("ballHeld ")
  IC14/1 -> ball2/3("robotIdx "), Display47/1
  ball2/2(ballHeld) -> [ballHeld5], Mux9/3, IC15/1
  IC13/1 -> [robotIdx5], Display48/1
  ball2/3(robotIdx) -> IC13/1, IC14/1
  Demux16/3 -> [KickPower5]
  Demux20/3 -> [rPose_theta5]
  Demux20/2 -> [rPose_y5]
  Demux20/1 -> [rPose_x5]
  Memory7/1 -> Demux20/1
  idx3 goal_range_angles2/3(goalLeft_angle) -> Mux9/6, Display53/1
  idx3 goal_range_angles2/2(goalRange) -> Mux9/5, Display52/1
  idx3 goal_range_angles2/1(goalRight_angle) -> Display51/1, Mux9/4
  ball2/1(y) -> Variable Selector7/1, Display54/1, Scope6/1
  Zero Pad Detections15/1(y) -> ball2/1(u), idx3 goal_range_angles2/1(u), "Object Detections [range, angle, label]4"/1, Scope7/1  "robotDetections"
  Demux17/2 -> Mux9/1
  Multi-Robot Lidar Sensor5/1 -> Multi-Robot Visualizer4/2
  Demux17/1 -> Mux9/2
  Variable Selector7/1 -> Demux17/1
  Object Detector4/1 -> Zero Pad Detections15/1(u)  "detections"
  Mux9/1 -> robot_actions5/1, Display49/1
  Generic Vehicle Simulation4/1 -> Multi-Robot Visualizer4/1, Display41/1, Object Detector4/1, Display44/1, Memory7/1  "pose"
  Demux16/2 -> Mux8/3
  Demux16/1 -> [ballVel5], Mux8/1
  robot_actions5/1 -> Demux16/1, Display46/1  "v"
  Ground4/1 -> Mux8/2
  Mux8/1 -> Generic Vehicle Simulation4/1
  Zero Pad Detections13/1(y) -> MATLAB Function4/1(u), Display50/1  "robotDetections"
  Robot Detector5/1 -> Zero Pad Detections13/1(u)
  [objPoses] -> Object Detector4/2
  [objPoses] -> Object Detector5/2
  Robot Detector6/1 -> Zero Pad Detections14/1(u)
  Zero Pad Detections14/1(y) -> MATLAB Function6/1(u), Display59/1  "robotDetections"
  Mux10/1 -> Generic Vehicle Simulation5/1
  Ground5/1 -> Mux10/2
  robot_actions6/1 -> Display55/1, Demux18/1  "v"
  Demux18/1 -> Mux10/1, [ballVel6]
  Demux18/2 -> Mux10/3
  Generic Vehicle Simulation5/1 -> Memory8/1, Display45/1, Object Detector5/1, Display43/1, Multi-Robot Visualizer5/1  "pose"
  Mux11/1 -> Display58/1, robot_actions6/1
  Object Detector5/1 -> Zero Pad Detections16/1(u)  "detections"
  Variable Selector8/1 -> Demux19/1
  Demux19/1 -> Mux11/2
  Multi-Robot Lidar Sensor6/1 -> Multi-Robot Visualizer5/2
  Demux19/2 -> Mux11/1
  Zero Pad Detections16/1(y) -> Scope9/1, "Object Detections [range, angle, label]5"/1, idx3 goal_range_angles5/1(u), ball5/1(u)  "robotDetections"
  ball5/1(y) -> Scope8/1, Display63/1, Variable Selector8/1
  idx3 goal_range_angles5/1(goalRight_angle) -> Mux11/4, Display60/1
  idx3 goal_range_angles5/2(goalRange) -> Mux11/5, Display61/1
  idx3 goal_range_angles5/3(goalLeft_angle) -> Mux11/6, Display62/1
  Memory8/1 -> Demux21/1
  Demux21/1 -> [rPose_x6]
  Demux21/2 -> [rPose_y6]
  Demux21/3 -> [rPose_theta6]
  Demux18/3 -> [KickPower6]
  ball5/3(robotIdx) -> IC17/1, IC16/1
  IC16/1 -> Display57/1, [robotIdx6]
  ball5/2(ballHeld) -> IC18/1, Mux11/3, [ballHeld6]
  IC17/1 -> Display56/1, ball5/3("robotIdx ")
  IC18/1 -> ball5/2("ballHeld ")
  [objPoses] -> Object Detector6/2
  Robot Detector7/1 -> Zero Pad Detections17/1(u)
  Zero Pad Detections17/1(y) -> Display70/1, MATLAB Function5/1(u)  "robotDetections"
  Mux12/1 -> Generic Vehicle Simulation6/1
  Ground6/1 -> Mux12/2
  robot_actions7/1 -> Display66/1, Demux22/1  "v"
  Demux22/1 -> Mux12/1, [ballVel7]
  Demux22/2 -> Mux12/3
  Generic Vehicle Simulation6/1 -> Memory9/1, Display65/1, Object Detector6/1, Display64/1, Multi-Robot Visualizer6/1  "pose"
  Mux13/1 -> Display69/1, robot_actions7/1
  Object Detector6/1 -> Zero Pad Detections18/1(u)  "detections"
  Variable Selector10/1 -> Demux23/1
  Demux23/1 -> Mux13/2
  Multi-Robot Lidar Sensor7/1 -> Multi-Robot Visualizer6/2
  Demux23/2 -> Mux13/1
  Zero Pad Detections18/1(y) -> Scope11/1, "Object Detections [range, angle, label]6"/1, idx3 goal_range_angles6/1(u), ball6/1(u)  "robotDetections"
  ball6/1(y) -> Scope10/1, Display74/1, Variable Selector10/1
  idx3 goal_range_angles6/1(goalRight_angle) -> Mux13/4, Display71/1
  idx3 goal_range_angles6/2(goalRange) -> Mux13/5, Display72/1
  idx3 goal_range_angles6/3(goalLeft_angle) -> Mux13/6, Display73/1
  Memory9/1 -> Demux24/1
  Demux24/1 -> [rPose_x7]
  Demux24/2 -> [rPose_y7]
  Demux24/3 -> [rPose_theta7]
  Demux22/3 -> [KickPower7]
  ball6/3(robotIdx) -> IC20/1, IC19/1
  IC19/1 -> Display68/1, [robotIdx7]
  ball6/2(ballHeld) -> IC21/1, Mux13/3, [ballHeld7]
  IC20/1 -> Display67/1, ball6/3("robotIdx ")
  IC21/1 -> ball6/2("ballHeld ")
  [rPose_x5] -> idx3 goal_range_angles2/2(rPose_x)
  [rPose_y5] -> idx3 goal_range_angles2/3(rPose_y)
  [rPose_x6] -> idx3 goal_range_angles5/2(rPose_x)
  [rPose_y6] -> idx3 goal_range_angles5/3(rPose_y)
  [rPose_x7] -> idx3 goal_range_angles6/2(rPose_x)
  [rPose_y7] -> idx3 goal_range_angles6/3(rPose_y)
  Chart3/3(Team1score) -> Display86/1
  Chart3/4(Team2score) -> Display87/1
  IC24/1 -> Display77/1, ball7/2("ballHeld ")
  IC23/1 -> ball7/3("robotIdx ")
  ball7/2(ballHeld) -> IC24/1, [ballHeld8], Mux15/3
  IC22/1 -> Display78/1, [robotIdx8]
  ball7/3(robotIdx) -> IC23/1, IC22/1
  Demux27/3 -> [KickPower8]
  Demux26/3 -> [rPose_theta8]
  Demux26/2 -> [rPose_y8]
  Demux26/1 -> [rPose_x8]
  Memory10/1 -> Demux26/1
  idx3 goal_range_angles7/3(goalLeft_angle) -> GoalLeftAngle4/1
  idx3 goal_range_angles7/2(goalRange) -> Mux15/4, Goal Range4/1
  idx3 goal_range_angles7/1(goalRight_angle) -> Display81/1
  ball7/1(y) -> Variable Selector11/1, Display82/1, Scope12/1
  Zero Pad Detections21/1(y) -> "Object Detections [range, angle, label]7"/1, ball7/1(u), idx3 goal_range_angles7/1(u), Scope13/1  "robotDetections"
  Demux28/2 -> Mux15/1
  Multi-Robot Lidar Sensor8/1 -> Multi-Robot Visualizer7/2
  Demux28/1 -> Mux15/2
  Variable Selector11/1 -> Demux28/1
  Object Detector7/1 -> Zero Pad Detections21/1(u)  "detections"
  Mux15/1 -> robot_actions8/1, Display75/1, Display79/1
  Generic Vehicle Simulation7/1 -> Multi-Robot Visualizer7/1, Display83/1, Object Detector7/1, Memory10/1, Display84/1  "pose"
  Demux27/2 -> Mux14/3
  Demux27/1 -> [ballVel8], Mux14/1
  robot_actions8/1 -> Demux27/1, Display76/1  "v"
  Ground7/1 -> Mux14/2
  Mux14/1 -> Generic Vehicle Simulation7/1
  Zero Pad Detections19/1(y) -> Variable Selector12/1, Display80/1  "robotDetections"
  Robot Detector8/1 -> Zero Pad Detections19/1(u)
  [objPoses] -> Object Detector7/2
  Demux29/2 -> [rdet_angle8]
  Demux29/1 -> [rdet_range8]
  [rdet_range8] -> Mux15/5
  [rdet_angle8] -> Mux15/6
  Variable Selector12/1 -> Demux29/1
  [ballPose_x] -> Mux15/7
  [teamHeld] -> Mux15/8
  [rPose_x4] -> idx3 goal_range_angles7/2(rPose_x)
  [rPose_y4] -> idx3 goal_range_angles7/3(rPose_y)
  [leftpoleangle2] -> Mux5/9
  [teamHeld] -> Mux9/7
  [teamHeld] -> Mux11/7
  [teamHeld] -> Mux13/7
  [rightpoleangle3] -> Mux17/9
  [rPose_y2] -> idx3 goal_range_angles8/3(rPose_y)
  [rPose_x2] -> idx3 goal_range_angles8/2(rPose_x)
  [teamHeld] -> Mux17/8
  [ballPose_x] -> Mux17/7
  Variable Selector14/1 -> Demux33/1
  [rdet_angle3] -> Mux17/6
  [rdet_range3] -> Mux17/5
  Demux33/1 -> [rdet_range3]
  Demux33/2 -> [rdet_angle3]
  [objPoses] -> Object Detector8/2
  Robot Detector9/1 -> Zero Pad Detections22/1(u)
  Zero Pad Detections22/1(y) -> Display92/1, Variable Selector14/1  "robotDetections"
  Mux16/1 -> Generic Vehicle Simulation8/1
  Ground8/1 -> Mux16/2
  robot_actions9/1 -> Display88/1, Demux31/1  "v"
  Demux31/1 -> Mux16/1, [ballVel3]
  Demux31/2 -> Mux16/3
  Generic Vehicle Simulation8/1 -> Display96/1, Memory11/1, Object Detector8/1, Display95/1, Multi-Robot Visualizer8/1  "pose"
  Mux17/1 -> Display91/1, Display85/1, robot_actions9/1
  Object Detector8/1 -> Zero Pad Detections24/1(u)  "detections"
  Variable Selector13/1 -> Demux32/1
  Demux32/1 -> Mux17/2
  Multi-Robot Lidar Sensor9/1 -> Multi-Robot Visualizer8/2
  Demux32/2 -> Mux17/1
  Zero Pad Detections24/1(y) -> Scope15/1, idx3 goal_range_angles8/1(u), ball8/1(u), "Object Detections [range, angle, label]8"/1  "robotDetections"
  ball8/1(y) -> Scope14/1, Display94/1, Variable Selector13/1
  idx3 goal_range_angles8/1(goalRight_angle) -> Display93/1, [rightpoleangle3]
  idx3 goal_range_angles8/2(goalRange) -> Goal Range5/1, Mux17/4
  idx3 goal_range_angles8/3(goalLeft_angle) -> GoalLeftAngle5/1
  Memory11/1 -> Demux30/1
  Demux30/1 -> [rPose_x3]
  Demux30/2 -> [rPose_y3]
  Demux30/3 -> [rPose_theta3]
  Demux31/3 -> [KickPower3]
  ball8/3(robotIdx) -> IC25/1, IC26/1
  IC25/1 -> [robotIdx3], Display90/1
  ball8/2(ballHeld) -> [ballHeld3], Mux17/3, IC27/1
  IC26/1 -> ball8/3("robotIdx ")
  IC27/1 -> ball8/2("ballHeld "), Display89/1
  [ballPose_y] -> Mux17/10
  [ballPose_y] -> Mux5/10
  [BALLHELD] -> MATLAB Function2/5("ballheld ")
  [interception2] -> Mux18/2
  [interception1] -> Mux18/1
  [interception3] -> Mux18/3
  [posession6] -> Mux19/2
  [posession5] -> Mux19/1
  [posession7] -> Mux19/3
  Mux18/1 -> MATLAB Function2/1(team1_interception)
  Mux19/1 -> MATLAB Function2/4(team2_possession)
  MATLAB Function2/1(ballheld) -> [BallHeld]
  [BallHeld] -> Chart3/1(ballHeld)
  MATLAB Function4/1(angle) -> [angle5]
  MATLAB Function4/2(range) -> [range5]
  [range5] -> Mux9/8
  [angle5] -> Mux9/9
  MATLAB Function5/2(range) -> [range7]
  MATLAB Function5/1(angle) -> [angle7]
  [range7] -> Mux13/8
  [angle7] -> Mux13/9
  MATLAB Function6/2(range) -> [range6]
  MATLAB Function6/1(angle) -> [angle6]
  [range6] -> Mux11/8
  [angle6] -> Mux11/9
  Mux20/1 -> MATLAB Function2/2(team2_interception)
  [interception5] -> Mux20/1
  [interception6] -> Mux20/2
  [interception7] -> Mux20/3
  [posession3] -> Mux21/3
  [posession1] -> Mux21/1
  [posession2] -> Mux21/2
  Mux21/1 -> MATLAB Function2/3(team1_possession)
  MATLAB Function3/1(Morale) -> ?
  MATLAB Function7/5(interception) -> [interception1]
  MATLAB Function7/6(posession) -> [posession1]
  MATLAB Function7/1(Morale) -> Memory12/1
  MATLAB Function7/2(Agg) -> Memory13/1
  MATLAB Function7/3(attack) -> Memory14/1
  MATLAB Function7/4(defense) -> Memory15/1
  Memory12/1 -> MATLAB Function7/1(Morale1)
  Memory13/1 -> MATLAB Function7/2(Agg1)
  Memory14/1 -> MATLAB Function7/3(attack1)
  Memory15/1 -> MATLAB Function7/4(defense1)
  MATLAB Function8/2(Agg) -> Memory17/1
  MATLAB Function8/6(posession) -> [posession3]
  MATLAB Function8/3(attack) -> Memory18/1
  Memory19/1 -> MATLAB Function8/4(defense1)
  MATLAB Function8/1(Morale) -> Memory16/1
  Memory16/1 -> MATLAB Function8/1(Morale1)
  Memory18/1 -> MATLAB Function8/3(attack1)
  MATLAB Function8/5(interception) -> [interception3]
  Memory17/1 -> MATLAB Function8/2(Agg1)
  MATLAB Function8/4(defense) -> Memory19/1
  MATLAB Function9/2(Agg) -> Memory21/1
  MATLAB Function9/6(posession) -> [posession2]
  MATLAB Function9/3(attack) -> Memory22/1
  Memory23/1 -> MATLAB Function9/4(defense1)
  MATLAB Function9/1(Morale) -> Memory20/1
  Memory20/1 -> MATLAB Function9/1(Morale1)
  Memory22/1 -> MATLAB Function9/3(attack1)
  MATLAB Function9/5(interception) -> [interception2]
  Memory21/1 -> MATLAB Function9/2(Agg1)
  MATLAB Function9/4(defense) -> Memory23/1
  MATLAB Function10/2(Agg) -> Memory25/1
  MATLAB Function10/6(posession) -> [posession5]
  MATLAB Function10/3(attack) -> Memory26/1
  Memory27/1 -> MATLAB Function10/4(defense1)
  MATLAB Function10/1(Morale) -> Memory24/1
  Memory24/1 -> MATLAB Function10/1(Morale1)
  Memory26/1 -> MATLAB Function10/3(attack1)
  MATLAB Function10/5(interception) -> [interception5]
  Memory25/1 -> MATLAB Function10/2(Agg1)
  MATLAB Function10/4(defense) -> Memory27/1
  MATLAB Function11/2(Agg) -> Memory29/1
  MATLAB Function11/6(posession) -> [posession6]
  MATLAB Function11/3(attack) -> Memory30/1
  Memory31/1 -> MATLAB Function11/4(defense1)
  MATLAB Function11/1(Morale) -> Memory28/1
  Memory28/1 -> MATLAB Function11/1(Morale1)
  Memory30/1 -> MATLAB Function11/3(attack1)
  MATLAB Function11/5(interception) -> [interceptio6]
  Memory29/1 -> MATLAB Function11/2(Agg1)
  MATLAB Function11/4(defense) -> Memory31/1
  MATLAB Function12/2(Agg) -> Memory33/1
  MATLAB Function12/6(posession) -> [posession7]
  MATLAB Function12/3(attack) -> Memory34/1
  Memory35/1 -> MATLAB Function12/4(defense1)
  MATLAB Function12/1(Morale) -> Memory32/1
  Memory32/1 -> MATLAB Function12/1(Morale1)
  Memory34/1 -> MATLAB Function12/3(attack1)
  MATLAB Function12/5(interception) -> [interception7]
  Memory33/1 -> MATLAB Function12/2(Agg1)
  MATLAB Function12/4(defense) -> Memory35/1
